simulink model "robot"  (Simulink 8.8)
settings: Solver=ode45  StartTime=0.0  StopTime=1.5  RelTol=1e-3  EnableMultiTasking=on
PreLoadFcn:
  | Factory
InitFcn:
  | Factory
values from neighbouring files (symbols this model uses):
  Amp1d = [1]    [DEFAULT (2).m]    (also in Robot (2).m = [8,1000]; Robot.m = [8,1000])
  Amp1n = [1]    [DEFAULT (2).m]    (also in Robot (2).m = [27.999999999999996,5000]; Robot.m = [27.999999999999996,5000])
  Amp2d = [1]    [DEFAULT (2).m]    (also in Robot (2).m = [8,1000]; Robot.m = [8,1000])
  Amp2n = [1]    [DEFAULT (2).m]    (also in Robot (2).m = [27.999999996,5000]; Robot.m = [27.999999996,5000])
  AmpSat1 = Big    [DEFAULT (2).m]    (also in Robot (2).m = 480; Robot.m = 480)
  AmpSat2 = Big    [DEFAULT (2).m]    (also in Robot (2).m = 480; Robot.m = 480)
  BackEMF1 = 0    [DEFAULT (2).m]    (also in Robot (2).m = 0.381971863421; Robot.m = 0.381971863421)
  BackEMF2 = 0    [DEFAULT (2).m]    (also in Robot (2).m = 0.381971863421; Robot.m = 0.381971863421)
  Elec1d = [1]    [DEFAULT (2).m]    (also in Robot (2).m = [0.001200000000000,0.075000000000000]; Robot.m = [0.001200000000000,0.075000000000000])
  Elec1n = [1]    [DEFAULT (2).m]    (also in Robot (2).m = 1; Robot.m = 1)
  Elec2d = [1]    [DEFAULT (2).m]    (also in Robot (2).m = [0.001200,0.0750000]; Robot.m = [0.001200,0.0750000])
  Elec2n = [1]    [DEFAULT (2).m]    (also in Robot (2).m = 1; Robot.m = 1)
  FB0 = 0    [DEFAULT (2).m]    (also in Robot (2).m = 1; Robot.m = 1)
  FB1 = 0    [DEFAULT (2).m]    (also in Robot (2).m = 1; Robot.m = 1)
  FB2 = 0    [DEFAULT (2).m]    (also in Robot (2).m = 1; Robot.m = 1)
  Gear1 = 1    [DEFAULT (2).m]    (also in Robot (2).m = 0.02; Robot.m = 0.02)
  Gear2 = 1    [DEFAULT (2).m]    (also in Robot (2).m = 0.2; Robot.m = 0.2)
  GR1 = 50    [CONSTANTS.m]
  GR2 = 5    [CONSTANTS.m]
  Grav = 0    [DEFAULT (2).m]    (also in Robot (2).m = 12.7098; Robot.m = 12.7098)
  JntMax0 = Big    [DEFAULT (2).m]    (also in Robot (2).m = QU0; Robot.m = QU0)
  JntMax1 = Big    [DEFAULT (2).m]    (also in Robot (2).m = 1.57079632679; Robot.m = 1.57079632679)
  JntMax2 = Big    [DEFAULT (2).m]    (also in Robot (2).m = 2.51327412287; Robot.m = 2.51327412287)
  JntMin0 = -Big    [DEFAULT (2).m]    (also in Robot (2).m = QL0; Robot.m = QL0)
  JntMin1 = -Big    [DEFAULT (2).m]    (also in Robot (2).m = -3.14159265359; Robot.m = -3.14159265359)
  JntMin2 = -Big    [DEFAULT (2).m]    (also in Robot (2).m = -2.51327412287; Robot.m = -2.51327412287)
  Mech0d = [1]    [DEFAULT (2).m]    (also in Robot (2).m = [95.780000,70]; Robot.m = [M0 B0])
  Mech0n = [1]    [DEFAULT (2).m]    (also in Robot (2).m = 3.4361; Robot.m = 3.4361)
  Mech1d = [1]    [DEFAULT (2).m]    (also in Robot (2).m = [0.1947 0.0021]; Robot.m = [0.1947 0.0021])
  Mech1n = [1]    [DEFAULT (2).m]    (also in Robot (2).m = 1; Robot.m = 1)
  Mech2d = [1]    [DEFAULT (2).m]    (also in Robot (2).m = [0.0193000000,7.150000e-04]; Robot.m = [0.0193000000,7.150000e-04])
  Mech2n = [1]    [DEFAULT (2).m]    (also in Robot (2).m = 1; Robot.m = 1)
  Pump0d = [1]    [DEFAULT (2).m]    (also in Robot (2).m = [1,100]; Robot.m = [1,100])
  Pump0n = [1]    [DEFAULT (2).m]    (also in Robot (2).m = 413685600; Robot.m = 413685600)
  Pump0sat = Big    [DEFAULT (2).m]    (also in Robot (2).m = 1034214; Robot.m = 1034214)
  TConst1 = 1    [DEFAULT (2).m]    (also in Robot (2).m = 5; Robot.m = 5)
  TConst2 = 1    [DEFAULT (2).m]    (also in Robot (2).m = 5; Robot.m = 5)
libraries: simulink x3, vrlib x1
settings Model: Creator=Leos  LastModifiedBy=Jeffrey
settings DataIOCC: LimitDataPoints=off
settings OptimizationCC: ExpressionDepthLimit=2147483647
settings DebuggingCC: SolverPrmCheckMsg=warning
settings ConfigComp: CovSFcnEnable=off

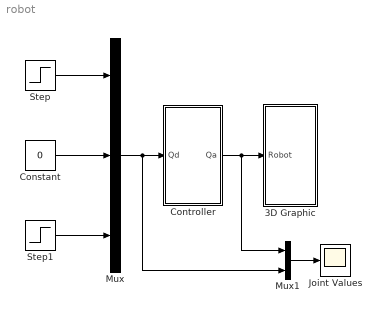
== system robot ==
  3D Graphic : Subsystem
  Constant : Constant  Value=0
  Controller : Subsystem
  Joint Values : Scope
  Mux : Mux  Inputs=3
  Mux1 : Mux  Inputs=2
  Step : Step  SampleTime=0
  Step1 : Step  Time=.5  Before=pi/2  After=0  SampleTime=0
  wires:
  Mux/1 -> Controller/1(Qd), Mux1/2
  Controller/1(Qa) -> Mux1/1, 3D Graphic/1(Robot)
  Mux1/1 -> Joint Values/1
  Constant/1 -> Mux/2
  Step/1 -> Mux/1
  Step1/1 -> Mux/3

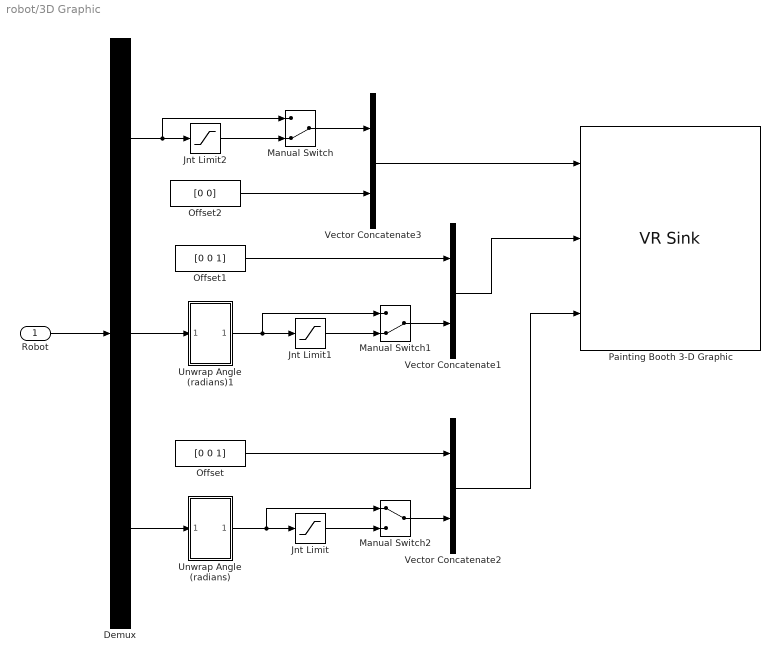
== system robot/3D Graphic ==
  Robot : Inport
  Demux : Demux  Outputs=3
  Jnt Limit : Saturate  UpperLimit=4*pi/5  LowerLimit=-4*pi/5
  Jnt Limit1 : Saturate  UpperLimit=pi/2  LowerLimit=-pi
  Jnt Limit2 : Saturate  UpperLimit=4.5  LowerLimit=-.5
  Manual Switch : ManualSwitch  CurrentSetting=0
  Manual Switch1 : ManualSwitch  CurrentSetting=0
  Manual Switch2 : ManualSwitch
  Offset : Constant  Value=[0 0 1]
  Offset1 : Constant  Value=[0 0 1]
  Offset2 : Constant  Value=[0 0]
  Painting Booth 3-D Graphic : vrlib/VR Sink  InstantiateOnLoad=on  SampleTime=-1  ViewEnable=on  RemoteChange=off  RemoteView=off  FieldsWritten=Q0.translation.3.1.1.double#Q1.rotation.4.1.1.double#Q2.rotation.4.1.1.double  WorldFileName=ROBOT.WRL  AutoView=on  VideoDimensions=[]  AllowVariableSize=off
  Unwrap Angle (radians) : Subsystem
  Unwrap Angle (radians)1 : Subsystem
  Vector Concatenate1 : Concatenate
  Vector Concatenate2 : Concatenate
  Vector Concatenate3 : Concatenate
  wires:
  Unwrap Angle (radians)/1(Out1) -> Manual Switch2/1, Jnt Limit/1
  Offset/1 -> Vector Concatenate2/1
  Unwrap Angle (radians)1/1(Out1) -> Manual Switch1/1, Jnt Limit1/1
  Offset1/1 -> Vector Concatenate1/1
  Offset2/1 -> Vector Concatenate3/2
  Robot/1 -> Demux/1
  Demux/1 -> Manual Switch/1, Jnt Limit2/1
  Demux/2 -> Unwrap Angle (radians)1/1(In1)
  Demux/3 -> Unwrap Angle (radians)/1(In1)
  Vector Concatenate3/1 -> Painting Booth 3-D Graphic/1
  Vector Concatenate1/1 -> Painting Booth 3-D Graphic/2
  Vector Concatenate2/1 -> Painting Booth 3-D Graphic/3
  Manual Switch/1 -> Vector Concatenate3/1
  Jnt Limit2/1 -> Manual Switch/2
  Manual Switch1/1 -> Vector Concatenate1/2
  Jnt Limit1/1 -> Manual Switch1/2
  Jnt Limit/1 -> Manual Switch2/2
  Manual Switch2/1 -> Vector Concatenate2/2

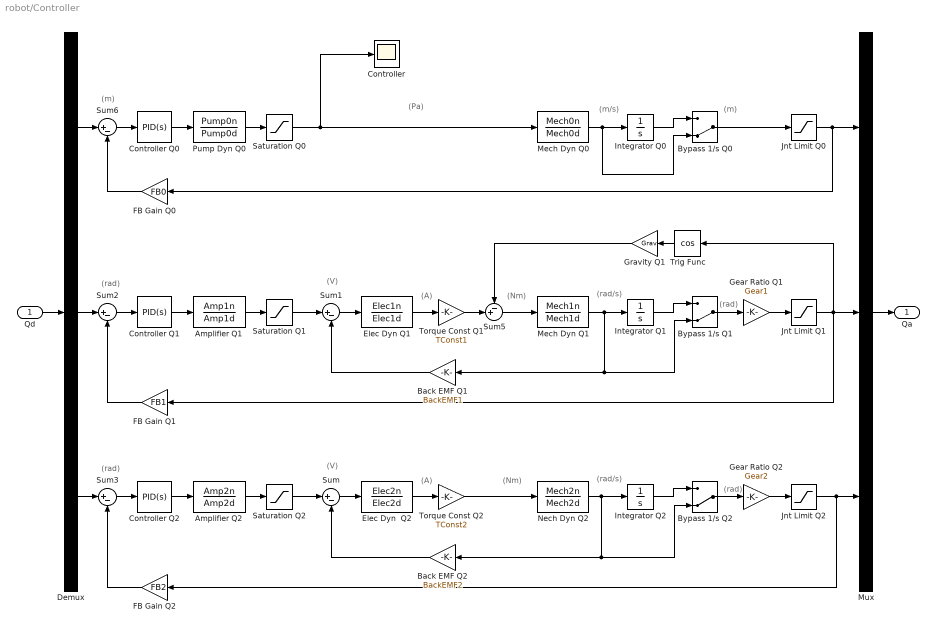
== system robot/Controller ==
  note: (rad)
  note: (V)
  note: (rad/s)
  note: (rad)
  note: (A)
  note: (Nm)
  note: (rad)
  note: (V)
  note: (rad/s)
  note: (rad)
  note: (A)
  note: (Nm)
  note: (m)
  note: (m)
  note: (Pa)
  note: (m/s)
  Qd : Inport
  Amplifier Q1 : TransferFcn  Numerator=Amp1n  Denominator=Amp1d
  Amplifier Q2 : TransferFcn  Numerator=Amp2n  Denominator=Amp2d
  Back EMF Q1 : Gain  Gain=BackEMF1
  Back EMF Q2 : Gain  Gain=BackEMF2
  Bypass 1/s Q0 : ManualSwitch  CurrentSetting=0
  Bypass 1/s Q1 : ManualSwitch  CurrentSetting=0
  Bypass 1/s Q2 : ManualSwitch  CurrentSetting=0
  Controller : Scope
  Controller Q0 : simulink/Continuous/PID Controller  Controller=PID  TimeDomain=Continuous-time  SampleTime=-1  IntegratorMethod=Forward Euler  FilterMethod=Forward Euler  Form=Parallel  UseFilter=on  ControllerParametersSource=internal  P=1.12859899259551e-07  I=7.12224648913286e-10  D=3.85340335553925e-06  N=24.0428525948039  InitialConditionSource=internal  InitialConditionForIntegrator=0  InitialConditionForFilter=0  ExternalReset=none  LimitOutput=off  UpperSaturationLimit=inf  LowerSaturationLimit=-inf  LinearizeAsGain=on  AntiWindupMode=none  Kb=1  TrackingMode=off  Kt=1  PParamMin=[]  PParamMax=[]  IParamMin=[]  IParamMax=[]  DParamMin=[]  DParamMax=[]  NParamMin=[]  NParamMax=[]  KbParamMin=[]  KbParamMax=[]  KtParamMin=[]  KtParamMax=[]  POutMin=[]  POutMax=[]  IOutMin=[]  IOutMax=[]  DOutMin=[]  DOutMax=[]  NOutMin=[]  NOutMax=[]  KbOutMin=[]  KbOutMax=[]  KtOutMin=[]  KtOutMax=[]  IntegratorOutMin=[]  IntegratorOutMax=[]  FilterOutMin=[]  FilterOutMax=[]  SumOutMin=[]  SumOutMax=[]  SumI1OutMin=[]  SumI1OutMax=[]  SumI2OutMin=[]  SumI2OutMax=[]  SumI3OutMin=[]  SumI3OutMax=[]  SumDOutMin=[]  SumDOutMax=[]  SaturationOutMin=[]  SaturationOutMax=[]  IntegratorContinuousStateAttributes=''  IntegratorStateMustResolveToSignalObject=off  IntegratorRTWStateStorageClass=Auto  FilterContinuousStateAttributes=''  FilterStateMustResolveToSignalObject=off  FilterRTWStateStorageClass=Auto  DifferentiatorICPrevScaledInput=0  DifferentiatorOutMin=[]  DifferentiatorOutMax=[]
  Controller Q1 : simulink/Continuous/PID Controller  Controller=PID  TimeDomain=Continuous-time  SampleTime=-1  IntegratorMethod=Forward Euler  FilterMethod=Forward Euler  Form=Parallel  UseFilter=on  ControllerParametersSource=internal  P=1226.04910924633  I=60998.3916220342  D=3.02160423589747  N=758303.123684934  InitialConditionSource=internal  InitialConditionForIntegrator=0  InitialConditionForFilter=0  ExternalReset=none  LimitOutput=off  UpperSaturationLimit=inf  LowerSaturationLimit=-inf  LinearizeAsGain=on  AntiWindupMode=none  Kb=1  TrackingMode=off  Kt=1  PParamMin=[]  PParamMax=[]  IParamMin=[]  IParamMax=[]  DParamMin=[]  DParamMax=[]  NParamMin=[]  NParamMax=[]  KbParamMin=[]  KbParamMax=[]  KtParamMin=[]  KtParamMax=[]  POutMin=[]  POutMax=[]  IOutMin=[]  IOutMax=[]  DOutMin=[]  DOutMax=[]  NOutMin=[]  NOutMax=[]  KbOutMin=[]  KbOutMax=[]  KtOutMin=[]  KtOutMax=[]  IntegratorOutMin=[]  IntegratorOutMax=[]  FilterOutMin=[]  FilterOutMax=[]  SumOutMin=[]  SumOutMax=[]  SumI1OutMin=[]  SumI1OutMax=[]  SumI2OutMin=[]  SumI2OutMax=[]  SumI3OutMin=[]  SumI3OutMax=[]  SumDOutMin=[]  SumDOutMax=[]  SaturationOutMin=[]  SaturationOutMax=[]  IntegratorContinuousStateAttributes=''  IntegratorStateMustResolveToSignalObject=off  IntegratorRTWStateStorageClass=Auto  FilterContinuousStateAttributes=''  FilterStateMustResolveToSignalObject=off  FilterRTWStateStorageClass=Auto  DifferentiatorICPrevScaledInput=0  DifferentiatorOutMin=[]  DifferentiatorOutMax=[]
  Controller Q2 : simulink/Continuous/PID Controller  Controller=PID  TimeDomain=Continuous-time  SampleTime=-1  IntegratorMethod=Forward Euler  FilterMethod=Forward Euler  Form=Parallel  UseFilter=on  ControllerParametersSource=internal  P=177.314254762784  I=66303.6754400911  D=0.0941138886063654  N=1639774.15634163  InitialConditionSource=internal  InitialConditionForIntegrator=0  InitialConditionForFilter=0  ExternalReset=none  LimitOutput=off  UpperSaturationLimit=inf  LowerSaturationLimit=-inf  LinearizeAsGain=on  AntiWindupMode=none  Kb=1  TrackingMode=off  Kt=1  PParamMin=[]  PParamMax=[]  IParamMin=[]  IParamMax=[]  DParamMin=[]  DParamMax=[]  NParamMin=[]  NParamMax=[]  KbParamMin=[]  KbParamMax=[]  KtParamMin=[]  KtParamMax=[]  POutMin=[]  POutMax=[]  IOutMin=[]  IOutMax=[]  DOutMin=[]  DOutMax=[]  NOutMin=[]  NOutMax=[]  KbOutMin=[]  KbOutMax=[]  KtOutMin=[]  KtOutMax=[]  IntegratorOutMin=[]  IntegratorOutMax=[]  FilterOutMin=[]  FilterOutMax=[]  SumOutMin=[]  SumOutMax=[]  SumI1OutMin=[]  SumI1OutMax=[]  SumI2OutMin=[]  SumI2OutMax=[]  SumI3OutMin=[]  SumI3OutMax=[]  SumDOutMin=[]  SumDOutMax=[]  SaturationOutMin=[]  SaturationOutMax=[]  IntegratorContinuousStateAttributes=''  IntegratorStateMustResolveToSignalObject=off  IntegratorRTWStateStorageClass=Auto  FilterContinuousStateAttributes=''  FilterStateMustResolveToSignalObject=off  FilterRTWStateStorageClass=Auto  DifferentiatorICPrevScaledInput=0  DifferentiatorOutMin=[]  DifferentiatorOutMax=[]
  Demux : Demux  Outputs=3
  Elec Dyn Q1 : TransferFcn  Numerator=Elec1n  Denominator=Elec1d
  Elec Dyn  Q2 : TransferFcn  Numerator=Elec2n  Denominator=Elec2d
  FB Gain Q0 : Gain  Gain=FB0
  FB Gain Q1 : Gain  Gain=FB1
  FB Gain Q2 : Gain  Gain=FB2
  Gear Ratio Q1 : Gain  Gain=Gear1
  Gear Ratio Q2 : Gain  Gain=Gear2
  Gravity Q1 : Gain  Gain=Grav
  Integrator Q0 : Integrator
  Integrator Q1 : Integrator  InitialCondition=-pi/2*GR1
  Integrator Q2 : Integrator  InitialCondition=pi/2*GR2
  Jnt Limit Q0 : Saturate  UpperLimit=JntMax0  LowerLimit=JntMin0
  Jnt Limit Q1 : Saturate  UpperLimit=JntMax1  LowerLimit=JntMin1
  Jnt Limit Q2 : Saturate  UpperLimit=JntMax2  LowerLimit=JntMin2
  Mech Dyn Q0 : TransferFcn  Numerator=Mech0n  Denominator=Mech0d
  Mech Dyn Q1 : TransferFcn  Numerator=Mech1n  Denominator=Mech1d
  Mux : Mux  Inputs=3
  Nech Dyn Q2 : TransferFcn  Numerator=Mech2n  Denominator=Mech2d
  Pump Dyn Q0 : TransferFcn  Numerator=Pump0n  Denominator=Pump0d
  Saturation Q0 : Saturate  UpperLimit=Pump0sat  LowerLimit=-Pump0sat
  Saturation Q1 : Saturate  UpperLimit=AmpSat1  LowerLimit=-AmpSat1
  Saturation Q2 : Saturate  UpperLimit=AmpSat2  LowerLimit=-AmpSat2
  Sum{,1..3,6} (5 alike) : Sum  Inputs=|+-
  Sum5 : Sum  Inputs=-+|
  Torque Const Q1 : Gain  Gain=TConst1
  Torque Const Q2 : Gain  Gain=TConst2
  Trig Func : Trigonometry  Operator=cos
  Qa : Outport
  wires:
  Qd/1 -> Demux/1
  Mux/1 -> Qa/1
  Controller Q2/1 -> Amplifier Q2/1
  Sum/1 -> Elec Dyn  Q2/1
  Sum3/1 -> Controller Q2/1
  Elec Dyn  Q2/1 -> Torque Const Q2/1
  Amplifier Q2/1 -> Saturation Q2/1
  Saturation Q2/1 -> Sum/1
  Back EMF Q2/1 -> Sum/2
  Torque Const Q2/1 -> Nech Dyn Q2/1
  Demux/3 -> Sum3/1
  FB Gain Q2/1 -> Sum3/2
  Nech Dyn Q2/1 -> Integrator Q2/1, Bypass 1/s Q2/2, Back EMF Q2/1
  Controller Q1/1 -> Amplifier Q1/1
  Sum1/1 -> Elec Dyn Q1/1
  Sum2/1 -> Controller Q1/1
  Elec Dyn Q1/1 -> Torque Const Q1/1
  Amplifier Q1/1 -> Saturation Q1/1
  Saturation Q1/1 -> Sum1/1
  Back EMF Q1/1 -> Sum1/2
  Demux/2 -> Sum2/1
  FB Gain Q1/1 -> Sum2/2
  Mech Dyn Q1/1 -> Integrator Q1/1, Bypass 1/s Q1/2, Back EMF Q1/1
  Torque Const Q1/1 -> Sum5/2
  Sum5/1 -> Mech Dyn Q1/1
  Controller Q0/1 -> Pump Dyn Q0/1
  Saturation Q0/1 -> Controller/1, Mech Dyn Q0/1
  Sum6/1 -> Controller Q0/1
  Pump Dyn Q0/1 -> Saturation Q0/1
  Demux/1 -> Sum6/1
  FB Gain Q0/1 -> Sum6/2
  Trig Func/1 -> Gravity Q1/1
  Gravity Q1/1 -> Sum5/1
  Bypass 1/s Q2/1 -> Gear Ratio Q2/1
  Bypass 1/s Q1/1 -> Gear Ratio Q1/1
  Integrator Q1/1 -> Bypass 1/s Q1/1
  Integrator Q2/1 -> Bypass 1/s Q2/1
  Integrator Q0/1 -> Bypass 1/s Q0/1
  Mech Dyn Q0/1 -> Bypass 1/s Q0/2, Integrator Q0/1
  Jnt Limit Q0/1 -> Mux/1, FB Gain Q0/1
  Bypass 1/s Q0/1 -> Jnt Limit Q0/1
  Gear Ratio Q1/1 -> Jnt Limit Q1/1
  Jnt Limit Q1/1 -> FB Gain Q1/1, Mux/2, Trig Func/1
  Gear Ratio Q2/1 -> Jnt Limit Q2/1
  Jnt Limit Q2/1 -> FB Gain Q2/1, Mux/3

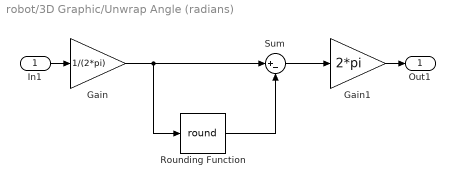
== system robot/3D Graphic/Unwrap Angle (radians) ==
  In1 : Inport
  Gain : Gain  Gain=1/(2*pi)
  Gain1 : Gain  Gain=2*pi
  Rounding Function : Rounding  Operator=round
  Sum : Sum  Inputs=|+-
  Out1 : Outport
  wires:
  Gain/1 -> Rounding Function/1, Sum/1
  Rounding Function/1 -> Sum/2
  Sum/1 -> Gain1/1
  In1/1 -> Gain/1
  Gain1/1 -> Out1/1

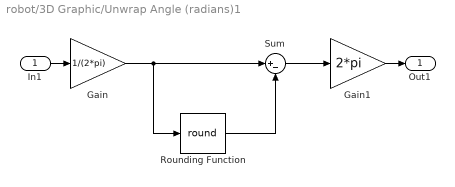
== system robot/3D Graphic/Unwrap Angle (radians)1 ==
  In1 : Inport
  Gain : Gain  Gain=1/(2*pi)
  Gain1 : Gain  Gain=2*pi
  Rounding Function : Rounding  Operator=round
  Sum : Sum  Inputs=|+-
  Out1 : Outport
  wires:
  Gain/1 -> Rounding Function/1, Sum/1
  Rounding Function/1 -> Sum/2
  Sum/1 -> Gain1/1
  In1/1 -> Gain/1
  Gain1/1 -> Out1/1
